simulink model "AM_modulated"  (R2013a)
settings: Solver=ode45  StartTime=0.0  StopTime=200.0  RelTol=1e-3
settings Model: Creator=root  LastModifiedBy=root

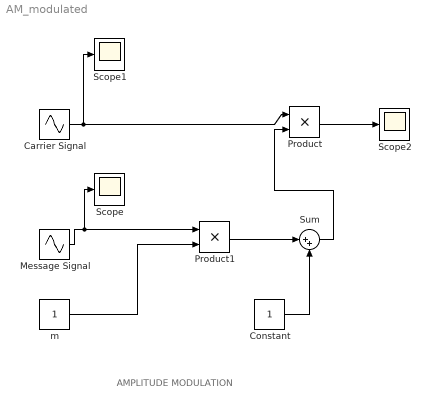
== system AM_modulated ==
  note: AMPLITUDE MODULATION
  Carrier Signal : Sin  Frequency=2*pi*25  SampleTime=1/5000
  Constant : Constant
  Message Signal : Sin  Frequency=2*pi  SampleTime=1/5000
  Product : Product
  Product1 : Product
  Scope : Scope
  Scope1 : Scope
  Scope2 : Scope
      settings: SaveName=ScopeData2
  Sum : Sum  Inputs=|++
  m : Constant
  wires:
  Carrier Signal/1 -> Scope1/1, Product/1
  Product/1 -> Scope2/1
  Message Signal/1 -> Scope/1, Product1/1
  Constant/1 -> Sum/2
  m/1 -> Product1/2
  Product1/1 -> Sum/1
  Sum/1 -> Product/2
